simulink model "State_space_Controller"  (R2020b)
settings: Solver=VariableStepAuto  StartTime=0.0  StopTime=50  RelTol=1e-3
libraries: simulink x1
settings Model: Creator=99003747  LastModifiedBy=99003747

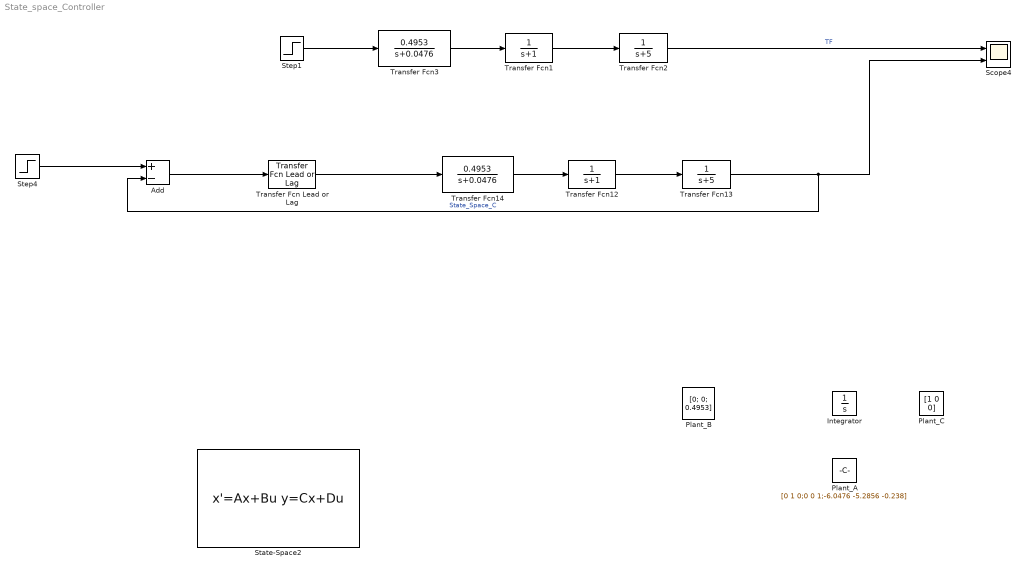
== system State_space_Controller ==
  Add : Sum  Inputs=+-
  Integrator : Integrator
  Plant_A : Constant  Value=[0 1 0;0 0 1;-6.0476 -5.2856 -0.238]
  Plant_B : Constant  Value=[0; 0; 0.4953]
  Plant_C : Constant  Value=[1 0 0]
  Scope4 : Scope  NumInputPorts=2
  State-Space2 : StateSpace  A=[0 1 0;0 0 1;-6.0476 -5.2856 -0.238]  B=[0;0;0.49533]  C=[1 0 0]  D=[0]  InitialCondition=0
  Step1 : Step  After=30  SampleTime=0
  Step4 : Step  After=30  SampleTime=0
  Transfer Fcn Lead or Lag : simulink/Discrete/Transfer Fcn Lead or Lag  PoleZ=0.95  ZeroZ=0.75  ICPrevOutput=0.0  ICPrevInput=0.0  DoSatur=off
      settings: SourceProductBaseCode=SL
  Transfer Fcn1 : TransferFcn  Denominator=[1 1]
  Transfer Fcn12 : TransferFcn  Denominator=[1 1]
  Transfer Fcn13 : TransferFcn  Denominator=[1 5]
  Transfer Fcn14 : TransferFcn  Numerator=[0.4953]  Denominator=[1 0.0476]
  Transfer Fcn2 : TransferFcn  Denominator=[1 5]
  Transfer Fcn3 : TransferFcn  Numerator=[0.4953]  Denominator=[1 0.0476]
  wires:
  Transfer Fcn12/1 -> Transfer Fcn13/1
  Transfer Fcn13/1 -> Add/2, Scope4/2  "State_Space_C"
  Transfer Fcn14/1 -> Transfer Fcn12/1
  Step4/1 -> Add/1
  Transfer Fcn1/1 -> Transfer Fcn2/1
  Transfer Fcn2/1 -> Scope4/1  "TF"
  Step1/1 -> Transfer Fcn3/1
  Transfer Fcn3/1 -> Transfer Fcn1/1
  Transfer Fcn Lead or Lag/1 -> Transfer Fcn14/1
  Add/1 -> Transfer Fcn Lead or Lag/1
